simulink model "Millsap_Justin_HW5_ARO4090"  (R2023b)
settings: Solver=VariableStepAuto  StartTime=0.0  StopTime=60  FixedStep=0.002  RelTol=1e-3  EnableMultiTasking=on
libraries: simulink_extras x4
settings Model: ExtModeTrigDuration=10000  Creator=jtmil  LastModifiedBy=jtmil
settings SolverCC: AlgebraicLoopSolver=TrustRegion  PositivePriorityOrder=on
settings DataIOCC: ReturnWorkspaceOutputs=off
settings OptimizationCC: LifeSpan=inf
settings DebuggingCC: UnconnectedInputMsg=warning  UnconnectedOutputMsg=warning  UnconnectedLineMsg=warning  ArithmeticOperatorsInVariantConditions=warning
settings ModelReferenceCC: EnableRefExpFcnMdlSchedulingChecks=on
settings SFSimCC: SimUseLocalCustomCode=off  CustomCodeUndefinedFunction=UseInterfaceOnly
settings RTWCC: Description=QUARC Win64 Target  SystemTargetFile=quarc_win64.tlc  TemplateMakefile=quarc_default_tmf  RTWUseLocalCustomCode=off
settings CodeAppCC: StateflowObjectComments=on
settings STFCustomTargetCC: TargetPreCompLibLocation=C:\PROGRA~3\QUARC\lib\2016a\win64\release  ConcurrentExecutionCompliant=on  GRTInterface=on  SystemTargetFile=quarc_win64.tlc
settings GRTTargetCC: TargetPreCompLibLocation=C:\PROGRA~3\QUARC\lib\2016a\win64\release  ParMdlRefBuildCompliant=off  CompOptLevelCompliant=off  CombineOutputUpdateFcns=off  MatFileLogging=off  CPPClassGenCompliant=off  GRTInterface=on  UseToolchainInfoCompliant=off  ExtMode=on  ExtModeMexFile=quarc_comm
settings ConfigComp: CovMetricSettings=dswe

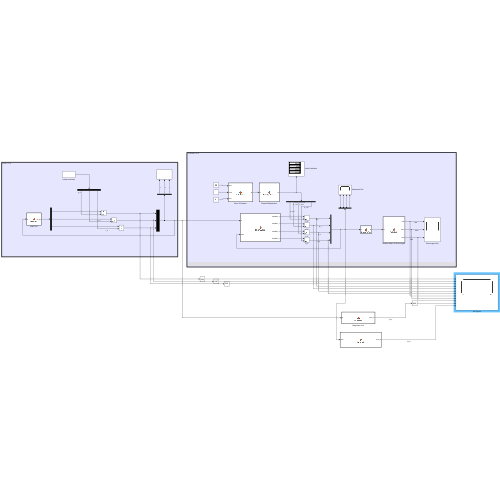
[thumbnail: Simulink's stored preview of the top-level diagram]
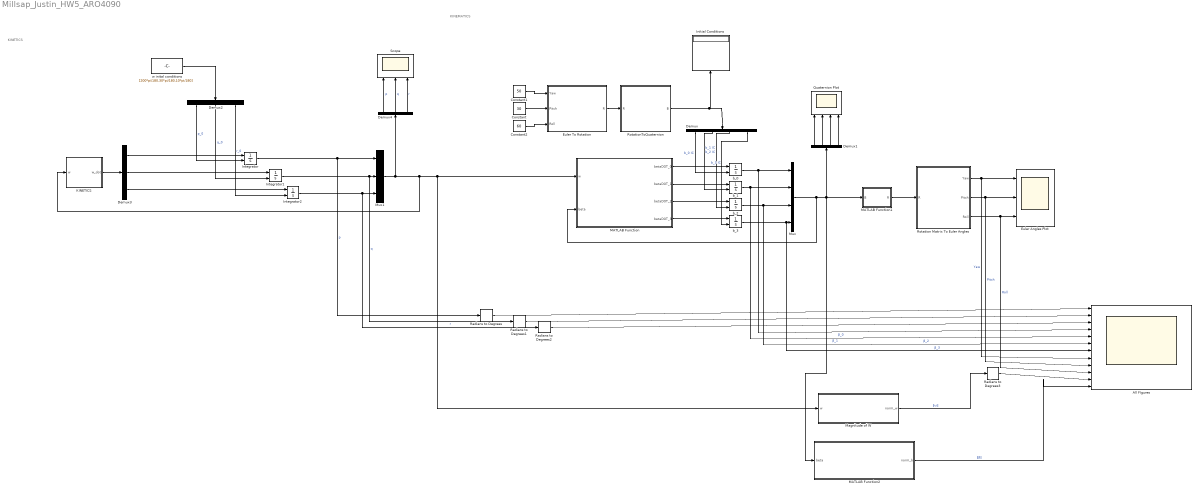
== system Millsap_Justin_HW5_ARO4090 ==
  note: KINETICS
  note: KINEMATICS
  All FIgures : Scope  NumInputPorts=12
  Constant : Constant  Value=30
  Constant1 : Constant  Value=50
  Constant2 : Constant  Value=60
  Demux : Demux
  Demux1 : Demux
  Demux2 : Demux  Outputs=3
  Demux3 : Demux  Outputs=3
  Demux4 : Demux  Outputs=3
  Euler Angles Plot : Scope  NumInputPorts=3
  Euler To Rotation : MATLAB Function  TreatAsAtomicUnit=on
  Initial Conditions : Display
  Integrator : Integrator  InitialConditionSource=external
  Integrator1 : Integrator  InitialConditionSource=external
  Integrator2 : Integrator  InitialConditionSource=external
  KINETICS : MATLAB Function  TreatAsAtomicUnit=on
  MATLAB Function : MATLAB Function  TreatAsAtomicUnit=on
  MATLAB Function1 : MATLAB Function  TreatAsAtomicUnit=on
  MATLAB Function2 : MATLAB Function  TreatAsAtomicUnit=on
  Magnitude of W : MATLAB Function  TreatAsAtomicUnit=on
  Mux : Mux
  Mux1 : Mux  Inputs=3
  Quaternion Plot : Scope  NumInputPorts=4
  Radians to Degrees{,1..3} (4 alike) : simulink_extras/Transformations/Radians to Degrees
  Rotation Matrix To Euler Angles : MATLAB Function  TreatAsAtomicUnit=on
  RotationToQuaternion : MATLAB Function  TreatAsAtomicUnit=on
  Scope : Scope  NumInputPorts=3
  b_{0..3} (4 alike) : Integrator  InitialConditionSource=external
  w inital conditions : Constant  Value=[200*pi/180,30*pi/180,10*pi/180]
  wires:
  Demux4/3 -> Scope/3  "r"
  Demux3/1 -> Integrator/1
  MATLAB Function1/1(R) -> Rotation Matrix To Euler Angles/1(R)
  Integrator2/1 -> Radians to Degrees2/1, Mux1/3  "r"
  MATLAB Function/2(betaDOT_1) -> b_1/1
  Integrator/1 -> Radians to Degrees/1, Mux1/1  "p"
  MATLAB Function/3(betaDOT_2) -> b_2/1
  Euler To Rotation/1(R) -> RotationToQuaternion/1(R)
  Demux2/3 -> Integrator2/2  "r_0"
  w inital conditions/1 -> Demux2/1
  Demux3/3 -> Integrator2/1
  Demux2/1 -> Integrator/2  "p_0"
  Integrator1/1 -> Radians to Degrees1/1, Mux1/2  "q"
  b_2/1 -> Mux/3, All FIgures/6  "β_2"
  Demux2/2 -> Integrator1/2  "q_0"
  Demux4/2 -> Scope/2  "q"
  Mux/1 -> MATLAB Function/2(beta), Demux1/1, MATLAB Function2/1(beta), MATLAB Function1/1(B)
  Demux1/2 -> Quaternion Plot/2
  b_1/1 -> Mux/2, All FIgures/5  "β_1"
  Mux1/1 -> Magnitude of W/1(w), MATLAB Function/1(w), KINETICS/1(w), Demux4/1
  Demux/3 -> b_2/2  "b_2 IC"
  Demux/4 -> b_3/2  "b_3 IC"
  Demux1/4 -> Quaternion Plot/4
  b_3/1 -> All FIgures/7, Mux/4  "β_3"
  b_0/1 -> Mux/1, All FIgures/4  "β_0"
  RotationToQuaternion/1(B) -> Initial Conditions/1, Demux/1
  Constant1/1 -> Euler To Rotation/1(Yaw)
  Demux/2 -> b_1/2  "b_1 IC"
  Demux/1 -> b_0/2  "b_0 IC"
  MATLAB Function/1(betaDOT_0) -> b_0/1
  Demux1/1 -> Quaternion Plot/1
  MATLAB Function/4(betaDOT_3) -> b_3/1
  Demux3/2 -> Integrator1/1
  Constant2/1 -> Euler To Rotation/3(Roll)
  Demux1/3 -> Quaternion Plot/3
  Constant/1 -> Euler To Rotation/2(Pitch)
  KINETICS/1(w_dot) -> Demux3/1
  Demux4/1 -> Scope/1  "p"
  Rotation Matrix To Euler Angles/1(Yaw) -> Euler Angles Plot/1, All FIgures/8  "Yaw"
  Rotation Matrix To Euler Angles/3(Roll) -> All FIgures/10, Euler Angles Plot/3  "Roll"
  Rotation Matrix To Euler Angles/2(Pitch) -> All FIgures/9, Euler Angles Plot/2  "Pitch"
  Magnitude of W/1(norm_w) -> Radians to Degrees3/1  "∥ω∥"
  MATLAB Function2/1(norm_b) -> All FIgures/12  "∥β∥"
  Radians to Degrees/1 -> All FIgures/1
  Radians to Degrees1/1 -> All FIgures/2
  Radians to Degrees2/1 -> All FIgures/3
  Radians to Degrees3/1 -> All FIgures/11

== matlab function Millsap_Justin_HW5_ARO4090/Magnitude of W ==
  data: w input; norm_w output
function norm_w = Magnitude(w)
norm_w = norm(w)
end

== matlab function Millsap_Justin_HW5_ARO4090/MATLAB Function ==
  data: w input; betaDOT_0 output; beta input; betaDOT_1 output; betaDOT_2 output; betaDOT_3 output
function [betaDOT_0 , betaDOT_1 , betaDOT_2 , betaDOT_3]= KINEMATICS(w , beta)


B_Beta = [-beta(2) -beta(3) -beta(4) ;
        beta(1) -beta(4) beta(3);
        beta(4) beta(1) -beta(2);
        -beta(3) beta(2) beta(1);]

beta_dot = 0.5*B_Beta*w

betaDOT_0 = beta_dot(1)
betaDOT_1 = beta_dot(2)
betaDOT_2 = beta_dot(3)
betaDOT_3 = beta_dot(4)



end

== matlab function Millsap_Justin_HW5_ARO4090/Euler To Rotation ==
  data: Yaw input; R output; Pitch input; Roll input
function R  = EulerToRot(Yaw,Pitch, Roll)

R1 = [ 1 0 0  ; 0 cosd(Roll) sind(Roll) ; 0 -sind(Roll) cosd(Roll)];
R2 = [cosd(Pitch) 0 -sind(Pitch); 0 1 0; sind(Pitch) 0 cosd(Pitch)];
R3 = [ cosd(Yaw) sind(Yaw) 0 ; -sind(Yaw) cosd(Yaw) 0 ; 0 0 1];

R = R1*R2*R3

end

== matlab function Millsap_Justin_HW5_ARO4090/Rotation Matrix To Euler Angles ==
  data: Yaw output; Pitch output; R input; Roll output
function [Yaw,Pitch,Roll] = RotToEuler(R)

Yaw = atan2d(R(1,2) , R(1,1)) % Yaw
Pitch = asind(-R(1,3))        % Pitch
Roll = atan2d(R(2,3),R(3,3))   % Roll

if Yaw<0
        Yaw=mod(Yaw+360,360);
    end

end

== matlab function Millsap_Justin_HW5_ARO4090/KINETICS ==
  data: w_dot output size=[3,1]; w input size=[3,1]
function w_dot = KINETICS(w)



% M = (10^-2)*[-6*w(1) ; 0 ; -5*w(3)];
M = (10^-2)*[-5 ; 0 ; 0];


rho = 1000;
l = 30*10^-2;

m = rho*l^3
I = zeros(3)
I(1,1) = (1/6)*m*l^2
I(2,2) = I(1,1)
I(3,3) = I(1,1)

I_B = I
w_skew = [ 0,     -w(3),  w(2);
           w(3),  0,     -w(1);
           -w(2),  w(1),  0];

w_dot = inv(I_B) * (M - w_skew*I_B*w)


end

== matlab function Millsap_Justin_HW5_ARO4090/RotationToQuaternion ==
  data: R input; B output
function B = RotToQuaternion(R)

B_0_check = (1/4)*(1 + R(1,1) + R(2,2) + R(3,3));
B_1_check = (1/4)*(1 + R(1,1) - R(2,2) - R(3,3));
B_2_check = (1/4)*(1 + R(2,2) - R(1,1) - R(3,3));
B_3_check = (1/4)*(1 + R(3,3) - R(1,1) - R(2,2));

B_check = [B_0_check ; B_1_check ; B_2_check ; B_3_check];

B_max = max(B_check);

% Initialize variables to ensure they are defined
B_0 = 0;
B_1 = 0;
B_2 = 0;
B_3 = 0;

if B_max == B_0_check % B_0 is max
    B_0 = sqrt(B_0_check);
    B_1 = (1/(4*B_0))*(R(2,3) - R(3,2));
    B_2 = (1/(4*B_0))*(R(3,1) - R(1,3));
    B_3 = (1/(4*B_0))*(R(1,2) - R(2,1));
elseif B_max == B_1_check % B_1 is max
    B_1 = sqrt(B_1_check);
    B_0 = (1/(4*B_1))*(R(2,3) - R(3,2));
    B_2 = (1/(4*B_1))*(R(1,2) - R(2,1));
    B_3 = (1/(4*B_1))*(R(3,1) - R(1,3));
elseif B_max == B_2_check % B_2 is max
    B_2 = sqrt(B_2_check);
    B_0 = (1/(4*B_2))*(R(3,1) - R(1,3));
    B_1 = (1/(4*B_2))*(R(1,2) + R(2,1));
    B_3 = (1/(4*B_2))*(R(2,3) + R(3,2));
elseif B_max == B_3_check % B_3 is max
    B_3 = sqrt(B_3_check);
    B_0 = (1/(4*B_3))*(R(1,2) - R(2,1));
    B_1 = (1/(4*B_3))*(R(3,1) + R(1,3));
    B_2 = (1/(4*B_3))*(R(2,3) + R(3,2));
end

B = [B_0 ; B_1 ; B_2 ; B_3];

if any(B < 0)
    B = -1*B;
end

end

== matlab function Millsap_Justin_HW5_ARO4090/MATLAB Function1 ==
  data: B input; R output
function R  = QuaterToRot(B)


R = [B(1)^2 + B(2)^2 - B(3)^2 - B(4)^2, 2*B(2)*B(3) + 2*B(1)*B(4), 2*B(2)*B(4) - 2*B(1)*B(3);
     2*B(2)*B(3) - 2*B(1)*B(4), B(1)^2 - B(2)^2 + B(3)^2 - B(4)^2, 2*B(3)*B(4) + 2*B(1)*B(2);
     2*B(2)*B(4) + 2*B(1)*B(3), 2*B(3)*B(4) - 2*B(1)*B(2), B(1)^2 - B(2)^2 - B(3)^2 + B(4)^2];



end

== matlab function Millsap_Justin_HW5_ARO4090/MATLAB Function2 ==
  data: beta input; norm_b output
function norm_b = Magnitude(beta)

norm_b = norm(beta)
end
